simulink model "automatas"  (R2018a)
settings: Solver=VariableStepAuto  StartTime=0.0  StopTime=10.0  RelTol=1e-3
values from neighbouring files (symbols this model uses):
  b_t = b_eq * r_t ^ 2 / R_w ^ 2    (= 27000)    [automatas_matlab.m]
  M_t = m_c + (J_w + J_m * r_t ^ 2)/ R_w ^ 2    (= 24008)    [automatas_matlab.m]
settings Model: Creator=gonzalo  LastModifiedBy=gonzalo

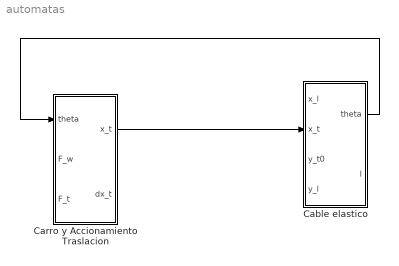
== system automatas ==
  Cable elastico : Subsystem
  Carro y Accionamiento Traslacion : Subsystem
  wires:
  Carro y Accionamiento Traslacion/1(x_t) -> Cable elastico/2(x_t)
  Cable elastico/1(theta) -> Carro y Accionamiento Traslacion/1(theta)

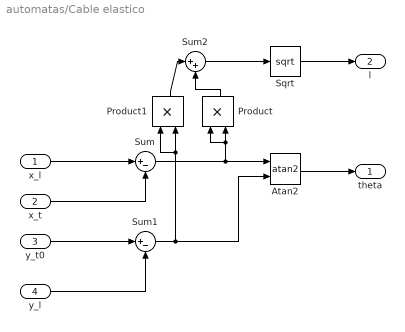
== system automatas/Cable elastico ==
  x_l : Inport
  x_t : Inport  Port=2
  y_t0 : Inport  Port=3
  y_l : Inport  Port=4
  Atan2 : Trigonometry  Operator=atan2
  Product : Product
  Product1 : Product
  Sqrt : Sqrt  SaturateOnIntegerOverflow=on
  Sum : Sum  Inputs=|+-
  Sum1 : Sum  Inputs=|+-
  Sum2 : Sum  Inputs=|++
  theta : Outport
  l : Outport  Port=2
  wires:
  x_l/1 -> Sum/1
  Sum1/1 -> Product1/1, Product1/2, Atan2/2
  Product/1 -> Sum2/2
  Atan2/1 -> theta/1
  Sum/1 -> Product/1, Product/2, Atan2/1
  y_l/1 -> Sum1/2
  Product1/1 -> Sum2/1
  Sum2/1 -> Sqrt/1
  Sqrt/1 -> l/1
  x_t/1 -> Sum/2
  y_t0/1 -> Sum1/1

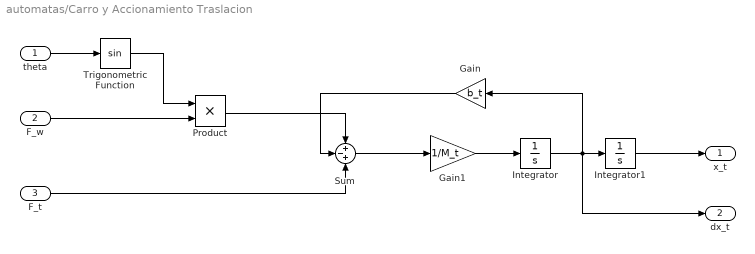
== system automatas/Carro y Accionamiento Traslacion ==
  theta : Inport
  F_w : Inport  Port=2
  F_t : Inport  Port=3
  Gain : Gain  Gain=b_t
  Gain1 : Gain  Gain=1/M_t
  Integrator : Integrator
  Integrator1 : Integrator
  Product : Product
  Sum : Sum  Inputs=+-+
  Trigonometric Function : Trigonometry
  x_t : Outport
  dx_t : Outport  Port=2
  wires:
  theta/1 -> Trigonometric Function/1
  F_t/1 -> Sum/3
  Product/1 -> Sum/1
  Gain/1 -> Sum/2
  Gain1/1 -> Integrator/1
  Integrator/1 -> dx_t/1, Gain/1, Integrator1/1
  Sum/1 -> Gain1/1
  Trigonometric Function/1 -> Product/1
  Integrator1/1 -> x_t/1
  F_w/1 -> Product/2
